simulink model "phase_detector_plus_pi_regulator"  (R2020b)
settings: Solver=VariableStepAuto  StartTime=0.0  StopTime=10.0  RelTol=1e-3
undefined symbols (not defined in the file or in its folder): f_rad, k_phi, ki, kp, Ts
settings Model: Creator=Kasper Laustsen  LastModifiedBy=Kasper Laustsen

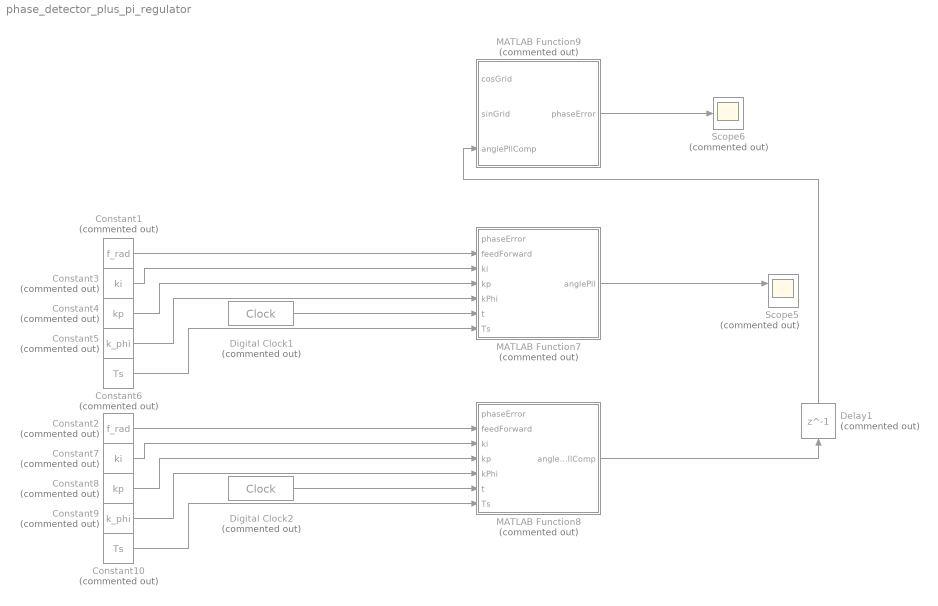
== system phase_detector_plus_pi_regulator ==
  Constant1 : Constant  Commented=on  Value=f_rad
  Constant10 : Constant  Commented=on  Value=Ts
  Constant2 : Constant  Commented=on  Value=f_rad
  Constant3 : Constant  Commented=on  Value=ki
  Constant4 : Constant  Commented=on  Value=kp
  Constant5 : Constant  Commented=on  Value=k_phi
  Constant6 : Constant  Commented=on  Value=Ts
  Constant7 : Constant  Commented=on  Value=ki
  Constant8 : Constant  Commented=on  Value=kp
  Constant9 : Constant  Commented=on  Value=k_phi
  Delay1 : Delay  Commented=on  DelayLength=1
  Digital Clock1 : DigitalClock  Commented=on  SampleTime=Ts
  Digital Clock2 : DigitalClock  Commented=on  SampleTime=Ts
  MATLAB Function7 : MATLAB Function  Commented=on  TreatAsAtomicUnit=on
  MATLAB Function8 : MATLAB Function  Commented=on  TreatAsAtomicUnit=on
  MATLAB Function9 : MATLAB Function  Commented=on  TreatAsAtomicUnit=on
  Scope5 : Scope  Commented=on  NumInputPorts=2
  Scope6 : Scope  Commented=on
  wires:
  Delay1/1 -> MATLAB Function9/3(anglePllComp)
  MATLAB Function9/1(phaseError) -> Scope6/1
  MATLAB Function8/1(anglePllComp) -> Delay1/1
  Constant2/1 -> MATLAB Function8/2(feedForward)
  Constant1/1 -> MATLAB Function7/2(feedForward)
  Digital Clock1/1 -> MATLAB Function7/6(t)
  Constant9/1 -> MATLAB Function8/5(kPhi)
  Digital Clock2/1 -> MATLAB Function8/6(t)
  Constant8/1 -> MATLAB Function8/4(kp)
  Constant6/1 -> MATLAB Function7/7(Ts)
  Constant7/1 -> MATLAB Function8/3(ki)
  Constant5/1 -> MATLAB Function7/5(kPhi)
  Constant10/1 -> MATLAB Function8/7(Ts)
  Constant4/1 -> MATLAB Function7/4(kp)
  Constant3/1 -> MATLAB Function7/3(ki)
  MATLAB Function7/1(anglePll) -> Scope5/1

== matlab function phase_detector_plus_pi_regulator/MATLAB Function7 ==
  data: phaseError input; anglePll output; feedForward input; ki input; kp input; kPhi input; t input; Ts input
function anglePll  = calling_pi_regulator(phaseError, feedForward, ki, kp, kPhi, t, Ts)
% coder.updateBuildInfo('addSourceFiles','abc_to_alphabeta.c');
% coder.cinclude('abc_to_alphabeta.h');
coder.updateBuildInfo('addSourceFiles','PLL.c');
coder.cinclude('PLL.h');

anglePll = 0.0;

anglePll = coder.ceval('pi_regulator', phaseError, feedForward, ki, kp, kPhi, t, Ts);

== matlab function phase_detector_plus_pi_regulator/MATLAB Function8 ==
  data: phaseError input; anglePllComp output; feedForward input; ki input; kp input; kPhi input; t input; Ts input
function anglePllComp  = calling_pi_regulator_comp(phaseError, feedForward, ki, kp, kPhi, t, Ts)
% coder.updateBuildInfo('addSourceFiles','abc_to_alphabeta.c');
% coder.cinclude('abc_to_alphabeta.h');
coder.updateBuildInfo('addSourceFiles','PLL.c');
coder.cinclude('PLL.h');

anglePllComp = 0.0;

anglePllComp = coder.ceval('pi_regulator_comp', phaseError, feedForward, ki, kp, kPhi, t, Ts);

== matlab function phase_detector_plus_pi_regulator/MATLAB Function9 ==
  data: cosGrid input; phaseError output; sinGrid input; anglePllComp input
function phaseError  = calling_phase_detector(cosGrid, sinGrid, anglePllComp)
% coder.updateBuildInfo('addSourceFiles','abc_to_alphabeta.c');
% coder.cinclude('abc_to_alphabeta.h');
coder.updateBuildInfo('addSourceFiles','PLL.c');
coder.cinclude('PLL.h');

phaseError = 0.0;

phaseError = coder.ceval('phase_detector', cosGrid, sinGrid, anglePllComp);
